simulink model "FCMW"  (R2024a)
settings: Solver=FixedStepAuto  StartTime=0.0  StopTime=inf  FixedStep=0.1
model workspace (MAT data in the model file):
  Ixx_values = 1.545e-05
  Iyy_values = 0.00073574
  Izz_values = 0.00074861
  base_link_Ixx = 7.46
  base_link_Iyy = 1.52
  base_link_Izz = 8.88
  base_link_mass = 19.0939
  gps0_Ixx = 2.1733e-06
  gps0_Iyy = 2.1733e-06
  gps0_Izz = 1.8e-07
  gps0_mass = 0.01
  i = 8
  imu_link_Ixx = 1e-05
  imu_link_Iyy = 1e-05
  imu_link_Izz = 1e-05
  imu_link_mass = 0.015
  masses = 0.085251
  phi = sym
  phi.s = 'symobj::fromString("eJytVL1OwzAQdpqWPwkhoaJCp0jwBIydCoKBEYoYWCyHmGLkOCXnlGbjKXgneCpst6LONQ0MjfTJzt35u+/uLIeEkBYhH59mbYdBxyzDPpl/odl3F3sTQ3YtoAQGIMbKmSv+c4t3LvIkmrJcsFjySLGUQ1QATyKhIijTLH69KtK0vEm40uJZ8Jz4OVuIs23xksnE2HteTL9mj/W6syAzjexbFqATKWKXe48sv30L4HpUphdSMOAwr/PEy/HtxQeIe9tiAoI+MFvY8MzTebo84/79vAcWc02DwfVskpmO4Vl8efFt9N9BfE6Hx+P7QgujEfOv1EF/J13xHVmsHeWSs1M7jyIGpP2wQYebFeVvBZPkr3429crn3LGATE65uwGV3jjfJQPxNOIa8fRQrKsn51ZZhd/hjlZ6gTV1US2+77hulkJpPnYdXs31uLlcrv6caZGp+rpu6eYejP9epKZHofniCJXw2UpeVyQ1iZkC6j0sliP0mhFEixXbgzX2+8X6AxDlhOk=", 2)'
  phi.Digits = 32
  rotors(1).mass = 0.085251
  rotors(1).Ixx = 1.545e-05
  rotors(1).Iyy = 0.00073574
  rotors(1).Izz = 0.00074861
  rotors(2).mass = 0.085251
  rotors(2).Ixx = 1.545e-05
  rotors(2).Iyy = 0.00073574
  rotors(2).Izz = 0.00074861
  rotors(3).mass = 0.085251
  rotors(3).Ixx = 1.545e-05
  rotors(3).Iyy = 0.00073574
  rotors(3).Izz = 0.00074861
  rotors(4).mass = 0.085251
  rotors(4).Ixx = 1.545e-05
  rotors(4).Iyy = 0.00073574
  rotors(4).Izz = 0.00074861
  rotors(5).mass = 0.085251
  rotors(5).Ixx = 1.545e-05
  rotors(5).Iyy = 0.00073574
  rotors(5).Izz = 0.00074861
  rotors(6).mass = 0.085251
  rotors(6).Ixx = 1.545e-05
  rotors(6).Iyy = 0.00073574
  rotors(6).Izz = 0.00074861
  rotors(7).mass = 0.085251
  rotors(7).Ixx = 1.545e-05
  rotors(7).Iyy = 0.00073574
  rotors(7).Izz = 0.00074861
  rotors(8).mass = 0.085251
  rotors(8).Ixx = 1.545e-05
  rotors(8).Iyy = 0.00073574
  rotors(8).Izz = 0.00074861
  theta = sym
  theta.s = 'symobj::fromString("eJytVL1OwzAQdpqWPwkhoaJCp0jwBIydCoKBESoxsFgOOYqR45ScU5qNp+CdylNhuxV13DQwNNInO3fn7767sxwSQlqEfH7ptR0GHb0M+2TxhXrfXe51DNk3wBIZIh9La674Lw0+gOdJNGU5Z7GASLIUMCoQkojLCMs0i99uijQt7xKQir9wyImbs+Vxtg1eM5Foe8+J6dfsfb32LIpMefYdA1SJ4LHNfUBW36EBghqV6ZXgDAEXdZ45Ob6d+MDj3jWYIKePzBQ2vHB0nq/O2H8375HBQtNgcDubZLpj/izmTnzb++94fFaHw+P6QgOt0edfq4P+TrriOzHYOMoVZ6d2HkWMnvbjBh12VhTeCybIX/1s6pXLuWeAmZiCvQGV3ljfNUP+PALl8fS8WFtPDkZZhd/igVZ64WvqerW4vtO6WXKpYGw7vJ7raXu5bP05UzyT9XXd0+09GP+9SE2PQvPF4TKB2VpeWyTViZlE6jwshiN0mhFEy9W3BxvssFx/ABFthPo=", 2)'
  theta.Digits = 32
  total_Ixx = 7.46
  total_Iyy = 1.53
  total_Izz = 8.89
  total_mass = 20
  total_rotor_Ixx = 0.0001236
  total_rotor_Iyy = 0.00588592
  total_rotor_Izz = 0.00598888
  total_rotor_masses = 0.682008
  u = sym
  u.s = 'symobj::fromString("eJytVL1OwzAQdpqWPwkhoaJCp0jwBIydCoKBESoxsFgOOYqR45ScU5qNp+CdylNhuxV13DQwNNInO3fn7767sxwSQlqEfH7ptR0GHb0M+2TxhXrfXe51DNk3wBIZIh9La674Lw0+gOdJNGU5Z7GASLIUMCoQkojLCMs0i99uijQt7xKQir9wyImbs+Vxtg1eM5Foe8+J6dfsfb32LIpMefYdA1SJ4LHNfUBW36EBghqV6ZXgDAEXdZ45Ob6d+MDj3jWYIKePzBQ2vHB0nq/O2H8375HBQtNgcDubZLpj/izmTnzb++94fFaHw+P6QgOt0edfq4P+TrriOzHYOMoVZ6d2HkWMnvbjBh12VhTeCybIX/1s6pXLuWeAmZiCvQGV3ljfNUP+PALl8fS8WFtPDkZZhd/igVZ64WvqerW4vtO6WXKpYGw7vJ7raXu5bP05UzyT9XXd0+09GP+9SE2PQvPF4TKB2VpeWyTViZlE6jwshiN0mhFEy9W3Bxvs0+X6AxH1hQs=", 2)'
  u.Digits = 32
  v = sym
  v.s = 'symobj::fromString("eJytVL1OwzAQdpqWPwkhoaJCp0jwBIydCoKBESoxsFgOOYqR45ScU5qNjTfgneCpsN2KOm4aGBrpk52783ff3VkOCSEtQt4/9doOg45ehn0y/0K97y72OobsGmCJDJGPpTVX/OcGb8DzJJqynLNYQCRZChgVCEnEZYRlmsUvV0WaljcJSMWfOOTEzdnyONsGz5lItL3nxPRr9r5eexZFpjz7lgGqRPDY5t4jy2/fAEGNyvRCcIaA8zpPnBzfTnzgcW8bTJDTe2YKG545Ok+XZ+y/m/fAYK5pMLieTTLdMX8WX0582/vveHxWh8Pj+kIDrdHnX6mD/k664jsyWDvKJWendh5FjJ72wwYddlYUXgsmyF/9bOqVy7ljgJmYgr0Bld5Y3yVD/jgC5fH0vFhbTw5GWYXf4o5WeuFr6nq1uL7jullyqWBsO7ya62FzuWz9OVM8k/V13dLNPRj/vUhNj0LzxeEygdlKXlsk1YmZROo8LIYjdJoRRIvVtwdr7B+L9QcSfYUc", 2)'
  v.Digits = 32
  w = sym
  w.s = 'symobj::fromString("eJytVL1OwzAQdpqWPwkhoaJCp0jwBIydCoKBESoxsFgOOYqR45ScU5qNp0C8EjwVtltRx00DQyN9snN3/u67O8shIaRFyPuHXtth0NHLsE/mX6j33cVex5BdAyyRIfKxtOaK/9zgDXieRFOWcxYLiCRLAaMCIYm4jLBMs/jlqkjT8iYBqfgTh5y4OVseZ9vgOROJtvecmH7N3tdrz6LIlGffMkCVCB7b3Htk+e0bIKhRmV4IzhBwXueJk+PbiQ887m2DCXJ6z0xhwzNH5+nyjP138x4YzDUNBtezSaY75s/iy4lve/8dj8/qcHhcX2igNfr8K3XQ30lXfEcGa0e55OzUzqOI0dN+2KDDzorCa8EE+aufTb1yOXcMMBNTsDeg0hvru2TIH0egPJ6eF2vrycEoq/Bb3NFKL3xNXa8W13dcN0suFYxth1dzPWwul60/Z4pnsr6uW7q5B+O/F6npUWi+OFwmMFvJa4ukOjGTSJ2HxXCETjOCaLH69mCN/XOx/gATBYUt", 2)'
  w.Digits = 32
  x = sym
  x.s = 'symobj::fromString("eJytVEtOwzAQdZqWn4SQUFGhq0hwApZdFQQLllCJBRvLIUMxcpyScUqz4xTcgaPAqbDdijpuGlg00pOdmfGbNzOWQ0JIi5D3D722w6Cjl2GfzL9Q77uLvY4huwZYIkPkY2nNFf+5wRvwPImmLOcsFhBJlgJGBUIScRlhmWbxy1WRpuVNAlLxJw45cXO2PM62wXMmEm3vOTH9mr2v155FkSnPvmWAKhE8trn3yPLbN0BQozK9EJwh4LzOEyfHtxMfeNzbBhPk9J6ZwoZnjs7T5Rn77+Y9MJhrGgyuZ5NMd8yfxZcT3/b+Ox6f1eHwuL7QQGv0+VfqoL+TrviODNaOcsnZqZ1HEaOn/bBBh50VhdeCCfJXP5t65XLuGGAmpmBvQKU31nfJkD+OQHk8PS/W1pODUVbht7ijlV74mrpeLa7vuG6WXCoY2w6v5nrYXC5bf84Uz2R9Xbd0cw/Gfy9S06PQfHG4TGC2ktcWSXViJpE6D4vhCJ1mBNFi9e3BGvvnYv0BE42FPg==", 2)'
  x.Digits = 32
  y = sym
  y.s = 'symobj::fromString("eJytVEtOwzAQdZqWn4SQUFGhq0hwApZdFQQLllCJBRvLIUMxcpyScUqz4xQchhvAqbDdijpuGlg00pOdmfGbNzOWQ0JIi5D3D722w6Cjl2GfzL9Q77uLvY4huwZYIkPkY2nNFf+5wRvwPImmLOcsFhBJlgJGBUIScRlhmWbxy1WRpuVNAlLxJw45cXO2PM62wXMmEm3vOTH9mr2v155FkSnPvmWAKhE8trn3yPLbN0BQozK9EJwh4LzOEyfHtxMfeNzbBhPk9J6ZwoZnjs7T5Rn77+Y9MJhrGgyuZ5NMd8yfxZcT3/b+Ox6f1eHwuL7QQGv0+VfqoL+TrviODNaOcsnZqZ1HEaOn/bBBh50VhdeCCfJXP5t65XLuGGAmpmBvQKU31nfJkD+OQHk8PS/W1pODUVbht7ijlV74mrpeLa7vuG6WXCoY2w6v5nrYXC5bf84Uz2R9Xbd0cw/Gfy9S06PQfHG4TGC2ktcWSXViJpE6D4vhCJ1mBNFi9e3BGvvnYv0BFBWFTw==", 2)'
  y.Digits = 32
  z = sym
  z.s = 'symobj::fromString("eJytVL1OwzAQdpqWPwkhoaJCp0jwBIydCoKBESoxsFgOOYqR45ScU5qNp+CdgJfCdivquGlgaKRPdu7O3313ZzkkhLQIef/QazsMOnoZ9sn8C/W+u9jrGLJrgCUyRD6W1lzxnxu8Ac+TaMpyzmIBkWQpYFQgJBGXEZZpFr9cFWla3iQgFX/ikBM3Z8vjbBs8ZyLR9p4T06/Z+3rtWRSZ8uxbBqgSwWObe48sv30DBDUq0wvBGQLO6zxxcnw58YHHvW0wQU7vmSlseOboPF2esf9u3gODuabB4Ho2yXTH/Fl8OvFt77/j8VkdDo/rCw20Rp9/pQ76O+mK78hg7SiXnJ3aeRQxetoPG3TYWVF4LZggf/WzqVcu544BZmIK9gZUemN9lwz54wiUx9PzYm09ORhlFX6LO1rpha+p69Xi+o7rZsmlgrHt8Gquh83lsvXnTPFM1td1Szf3YPz3IjU9Cs0Xh8sEZit5bZFUJ2YSqfOwGI7QaUYQLVbfHqyxfy/WHxSdhWA=", 2)'
  z.Digits = 32
undefined symbols (not defined in the file or in its folder): rad, s
libraries: robotlib x13, simulink x7, aerolibconvert2 x1, sharedtransform x1
settings Model: PacingRate=50  Creator=hmcl  LastModifiedBy=hmcl
settings OptimizationCC: EnhancedBackFolding=on  PassReuseOutputArgsAs=Individual arguments  ZeroExternalMemoryAtStartup=off  ZeroInternalMemoryAtStartup=off  MaxStackSize=64  OptimizeBlockOrder=speed  DifferentSizesBufferReuse=on  OptimizationCustomize=off  EfficientTunableParamExpr=on
settings DebuggingCC: ParameterTunabilityLossMsg=error
settings HardwareCC: ProdBitPerPointer=32  ProdBitPerSizeT=32  ProdBitPerPtrDiffT=32  ProdLargestAtomicFloat=None  ProdIntDivRoundTo=Undefined  ProdEndianess=Unspecified  ProdWordSize=32  ProdHWDeviceType=Generic->Unspecified (assume 32-bit Generic)
settings SFSimCC: MATLABDynamicMemAlloc=off
settings RTWCC: Description=Embedded Coder  SystemTargetFile=ert.tlc  HardwareBoard=Robot Operating System (ROS)  TLCOptions="-aInlineSetEventsForThisBaseRateFcn=TLC_FALSE -aSuppressMultiTaskScheduler=TLC_FALSE  -aRateBasedStepFcn=0"  TemplateMakefile=ert_default_tmf  Toolchain=Catkin  TargetLang=C++  GPUComputeCapability=3.5
settings CodeAppCC: ForceParamTrailComments=on  IgnoreCustomStorageClasses=off  OperatorAnnotations=on  SimulinkDataObjDesc=on  SFDataObjDesc=on  InsertBlockDesc=on
settings ERTTargetCC: ERTCustomFileTemplate=rostime_codertarget_file_process.tlc

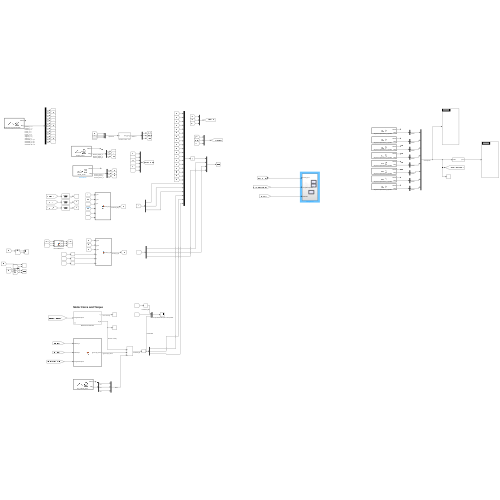
[thumbnail: Simulink's stored preview of the top-level diagram]
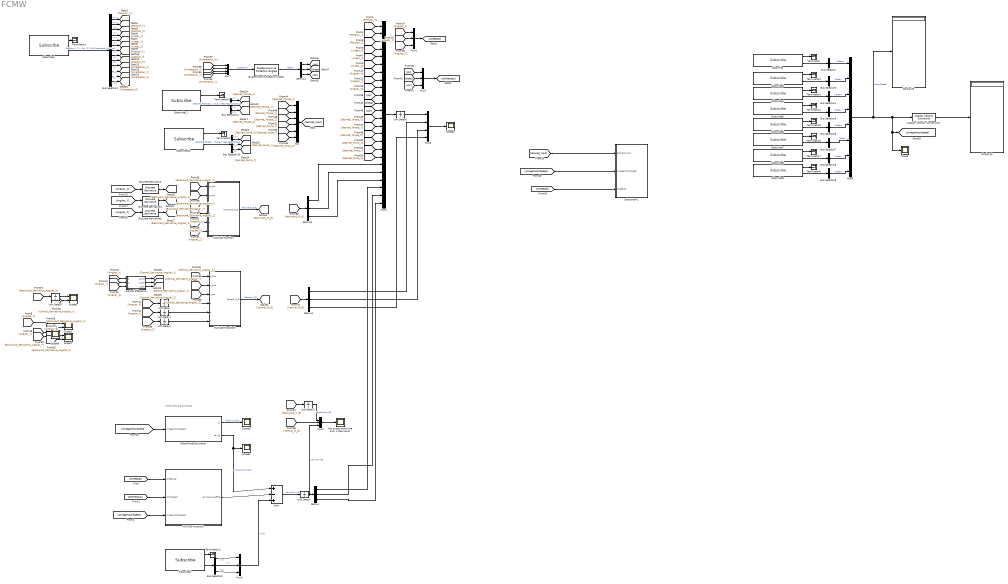
== system FCMW ==
  note: Motor Force and Torque
  Angular Velocity Conversion1 : aerolibconvert2/Angular Velocity Conversion  IU=rad/s  OU=rpm
  Bus Selector{,3..9} (8 alike) : BusSelector  OutputSignals=Data
  Bus Selector1 : BusSelector  OutputSignals=Pose.Pose.Position.X,Pose.Pose.Position.Y,Pose.Pose.Position.Z,Twist.Twist.Linear.X,Twist.Twist.Linear.Y,Twist.Twist.Linear.Z,Twist.Twist.Angular.X,Twist.Twist.Angular.Y,Twist.Twist.Angular.Z,Pose.Pose.Orientation.X,Pose.Pose.Orientation.Y,Pose.Pose.Orientation.Z,Pose.Pose.Orientation.W
  Bus Selector10 : BusSelector  OutputSignals=X,Y,Z
  Bus Selector11 : BusSelector  OutputSignals=X,Y,Z
  Bus Selector2 : BusSelector  OutputSignals=X,Y,Z
  Demux{,1,4..5} (4 alike) : Demux  Outputs=3
  Discrete Derivative : simulink/Discrete/Discrete Derivative  gainval=1  ICPrevScaledInput=0.0  OutMin=[]  OutMax=[]  OutDataType=fixdt(1, 16)  OutScaling=2^-10  DoSatur=off
  Discrete Derivative1 : simulink/Discrete/Discrete Derivative  gainval=1  ICPrevScaledInput=0.0  OutMin=[]  OutMax=[]  OutDataType=fixdt(1, 16)  OutScaling=2^-10  DoSatur=off
  Discrete Derivative2 : simulink/Discrete/Discrete Derivative  gainval=1  ICPrevScaledInput=0.0  OutMin=[]  OutMax=[]  OutDataType=fixdt(1, 16)  OutScaling=2^-10  DoSatur=off
  Display24 : Display
  Display25 : Display
  MATLAB Function : MATLAB Function  TreatAsAtomicUnit=on
  MATLAB Function1 : MATLAB Function  TreatAsAtomicUnit=on
  MATLAB Function3 : MATLAB Function  TreatAsAtomicUnit=on
  MotorForceCalculation : Subsystem  mask{b=0.00053, d=0.0000169, L1=0.545, L2=0.36, L3=1.08}
      mask prompts: b "b = motorConstant [N*s^2/rad^2] ="; d "d = momentConstant [N*m*s^2/rad^2] ="; L1 "L1 ="; L2 "L2 ="; L3 "L3 ="
  Mux : Mux  Inputs=6
  Mux{1..4} (4 alike) : Mux  Inputs=3
  Mux5 : Mux  Inputs=24
  Mux6 : Mux
  Mux7 : Mux
  Mux9 : Mux  Inputs=8
  Quaternions to Rotation Angles : sharedtransform/Quaternions to Rotation Angles  rotationOrder=ZYX  aMode=aMode
  Scope{,2..4} (4 alike) : Scope
  Scope{1,5..7} (4 alike) : Scope  NumInputPorts=2
  Subscribe : robotlib/Subscribe  topicSource=Select from ROS network  topic=/my/octocopter3/motor_speed/0  messageType=std_msgs/Float64  SampleTime=-1  legacyBusStruct=off  messageQueueLength=1
  Subscribe1 : robotlib/Subscribe  topicSource=Select from ROS network  topic=/mavros/local_position/odom  messageType=nav_msgs/Odometry  SampleTime=-1  legacyBusStruct=off  messageQueueLength=1
  Subscribe10 : robotlib/Subscribe  topicSource=Select from ROS network  topic=/thrust_vector  messageType=geometry_msgs/Vector3  SampleTime=-1  legacyBusStruct=off  messageQueueLength=1
  Subscribe11 : robotlib/Subscribe  topicSource=Select from ROS network  topic=/torque_vector  messageType=geometry_msgs/Vector3  SampleTime=-1  legacyBusStruct=off  messageQueueLength=1
  Subscribe2 : robotlib/Subscribe  topicSource=Select from ROS network  topic=/my_custom_wind  messageType=geometry_msgs/Vector3  SampleTime=-1  legacyBusStruct=off  messageQueueLength=1
  Subscribe3 : robotlib/Subscribe  topicSource=Select from ROS network  topic=/my/octocopter3/motor_speed/1  messageType=std_msgs/Float64  SampleTime=-1  legacyBusStruct=off  messageQueueLength=1
  Subscribe4 : robotlib/Subscribe  topicSource=Select from ROS network  topic=/my/octocopter3/motor_speed/2  messageType=std_msgs/Float64  SampleTime=-1  legacyBusStruct=off  messageQueueLength=1
  Subscribe5 : robotlib/Subscribe  topicSource=Select from ROS network  topic=/my/octocopter3/motor_speed/3  messageType=std_msgs/Float64  SampleTime=-1  legacyBusStruct=off  messageQueueLength=1
  Subscribe6 : robotlib/Subscribe  topicSource=Select from ROS network  topic=/my/octocopter3/motor_speed/4  messageType=std_msgs/Float64  SampleTime=-1  legacyBusStruct=off  messageQueueLength=1
  Subscribe7 : robotlib/Subscribe  topicSource=Select from ROS network  topic=/my/octocopter3/motor_speed/5  messageType=std_msgs/Float64  SampleTime=-1  legacyBusStruct=off  messageQueueLength=1
  Subscribe8 : robotlib/Subscribe  topicSource=Select from ROS network  topic=/my/octocopter3/motor_speed/6  messageType=std_msgs/Float64  SampleTime=-1  legacyBusStruct=off  messageQueueLength=1
  Subscribe9 : robotlib/Subscribe  topicSource=Select from ROS network  topic=/my/octocopter3/motor_speed/7  messageType=std_msgs/Float64  SampleTime=-1  legacyBusStruct=off  messageQueueLength=1
  Subsystem2 : Subsystem
  Sum : Sum  Inputs=|+-+
  Terminator{,1..11} (12 alike) : Terminator
  Unit Delay{,1..6} (7 alike) : UnitDelay  SampleTime=-1  HasFrameUpgradeWarning=on
  central difference : MATLAB Function  TreatAsAtomicUnit=on
  this scope shows the prior 1 step result : Scope
  wires:
  Mux7/1 -> Quaternions to Rotation Angles/1  "quertanion"
  Subscribe1/2 -> Bus Selector1/1  "Position_X = x  Position_Y = y Position_Z = z Linear_X = u Linear_Y = v Linear_Z = w Angular_X = p Angular_Y = q Angular_Z = r Orientation_X = q1  Orientation_Y = q2 Orientation_Z = q3 Orientation_W = q4"
  Subscribe1/1 -> Terminator1/1
  Subscribe/1 -> Terminator/1
  Subscribe3/1 -> Terminator2/1
  Subscribe4/1 -> Terminator3/1
  Subscribe5/1 -> Terminator4/1
  Subscribe6/1 -> Terminator5/1
  Subscribe7/1 -> Terminator6/1
  Subscribe8/1 -> Terminator7/1
  Subscribe9/1 -> Terminator8/1
  Subscribe/2 -> Bus Selector/1
  Subscribe3/2 -> Bus Selector3/1
  Subscribe4/2 -> Bus Selector4/1
  Subscribe5/2 -> Bus Selector5/1
  Subscribe6/2 -> Bus Selector6/1
  Subscribe7/2 -> Bus Selector7/1
  Subscribe8/2 -> Bus Selector8/1
  Subscribe9/2 -> Bus Selector9/1
  Mux9/1 -> Display25/1, Angular Velocity Conversion1/1, Scope/1, [omegaMotorSpeed]  "motorSpeed"
  Bus Selector/1 -> Mux9/1  "<Data>"
  Bus Selector3/1 -> Mux9/2  "<Data>"
  Bus Selector4/1 -> Mux9/3  "<Data>"
  Bus Selector5/1 -> Mux9/4  "<Data>"
  Bus Selector6/1 -> Mux9/5  "<Data>"
  Bus Selector7/1 -> Mux9/6  "<Data>"
  Bus Selector8/1 -> Mux9/7  "<Data>"
  Bus Selector9/1 -> Mux9/8  "<Data>"
  [desired_input] -> Subsystem2/1(desired_input)
  [omegaMotorSpeed] -> Subsystem2/2(omegaMotorSpeed)
  [OMEGAB] -> Subsystem2/3(OMEGAB)
  Angular Velocity Conversion1/1 -> Display24/1
  Mux5/1 -> Unit Delay6/1
  Subscribe10/1 -> Terminator9/1
  Subscribe11/1 -> Terminator10/1
  Subscribe10/2 -> Bus Selector10/1  "Desired_Force_X Desired_Force_Y Desired_Force_Z"
  Subscribe11/2 -> Bus Selector11/1  "Desired_Torque_X Desired_Torque_Y Desired_Torque_Z"
  Demux5/1 -> Mux5/19
  Demux5/2 -> Mux5/20
  Demux5/3 -> Mux5/21
  Mux/1 -> [desired_input]
  Mux1/1 -> [OMEGAB]
  [omegaMotorSpeed] -> MotorForceCalculation/1(omegaMotorSpeed)
  [OMEGAB] -> MATLAB Function1/1(OMEGA_B)
  Mux2/1 -> [phithetapsi]
  [phithetapsi] -> MATLAB Function1/2(phithetapsi)
  [omegaMotorSpeed] -> MATLAB Function1/3(omegaMotorSpeed)
  Subscribe2/1 -> Terminator11/1
  Subscribe2/2 -> Bus Selector2/1
  MATLAB Function1/1(gyroscopic_effect) -> Sum/2
  MotorForceCalculation/2(tau_B) -> Scope4/1, Sum/1  "moment on body"
  Bus Selector2/1 -> Mux3/1  "<X>"
  Bus Selector2/2 -> Mux3/2  "<Y>"
  Bus Selector2/3 -> Mux3/3  "<Z>"
  Mux3/1 -> Sum/3  "wind"
  MotorForceCalculation/1(f_t) -> Scope3/1  "force on body"
  Sum/1 -> Unit Delay4/1  "nominal M_B"
  Mux4/1 -> this scope shows the prior 1 step result/1
  Unit Delay/1 -> MATLAB Function3/4(p)
  Unit Delay1/1 -> MATLAB Function3/5(q)
  Unit Delay2/1 -> MATLAB Function3/6(r)
  Unit Delay3/1 -> Mux4/1  "backward_MB"
  Unit Delay5/1 -> Scope5/1
  Unit Delay4/1 -> Mux4/3, Demux/1  "nominal MB"
  Demux/1 -> Mux5/22
  Demux/2 -> Mux5/23
  Demux/3 -> Mux5/24
  Unit Delay6/1 -> Mux6/1
  Mux6/1 -> Scope2/1
  Demux1/1 -> Mux6/2
  Demux1/2 -> Mux6/3
  Demux1/3 -> Mux6/4
  Bus Selector1/1 -> [Position_X]  "<X>"
  [Position_X] -> Mux5/1
  Bus Selector1/2 -> [Position_Y]  "<Y>"
  [Position_Y] -> Mux5/2
  Bus Selector1/3 -> [Position_Z]  "<Z>"
  [Position_Z] -> Mux5/3
  Bus Selector1/4 -> [Linear_X]  "<X>"
  [Linear_X] -> Mux5/4
  Bus Selector1/5 -> [Linear_Y]  "<Y>"
  [Linear_Y] -> Mux5/5
  Bus Selector1/6 -> [Linear_Z]  "<Z>"
  [Linear_Z] -> Mux5/6
  Bus Selector1/7 -> [Angular_X]  "<X>"
  [Angular_X] -> Scope1/1
  [Angular_X] -> central difference/1(p)
  [Angular_X] -> Unit Delay/1
  [Angular_X] -> Mux5/7
  [Angular_X] -> Mux1/1
  [Angular_X] -> Discrete Derivative/1
  [Angular_X] -> MATLAB Function/4(p)
  Bus Selector1/8 -> [Angular_Y]  "<Y>"
  [Angular_Y] -> Discrete Derivative1/1
  [Angular_Y] -> Scope6/1
  [Angular_Y] -> MATLAB Function/5(q)
  [Angular_Y] -> Unit Delay1/1
  [Angular_Y] -> Mux5/8
  [Angular_Y] -> Mux1/2
  [Angular_Y] -> central difference/2(q)
  Bus Selector1/9 -> [Angular_Z]  "<Z>"
  [Angular_Z] -> Mux1/3
  [Angular_Z] -> Discrete Derivative2/1
  [Angular_Z] -> Scope7/1
  [Angular_Z] -> Mux5/9
  [Angular_Z] -> MATLAB Function/6(r)
  [Angular_Z] -> central difference/3(r)
  [Angular_Z] -> Unit Delay2/1
  Bus Selector1/10 -> [Orientation_X]  "<X>"
  [Orientation_X] -> Mux7/4
  Bus Selector1/11 -> [Orientation_Y]  "<Y>"
  [Orientation_Y] -> Mux7/3
  Bus Selector1/12 -> [Orientation_Z]  "<Z>"
  [Orientation_Z] -> Mux7/2
  Bus Selector1/13 -> [Orientation_W]  "<W>"
  [Orientation_W] -> Mux7/1
  Quaternions to Rotation Angles/1 -> Demux4/1  "radian"
  Demux4/1 -> [phi]
  [phi] -> Mux5/10
  [phi] -> Mux2/1
  Demux4/2 -> [theta]
  [theta] -> Mux5/11
  [theta] -> Mux2/2
  Demux4/3 -> [psi]
  [psi] -> Mux2/3
  [psi] -> Mux5/12
  Bus Selector11/1 -> [Desired_Torque_X]  "<X>"
  [Desired_Torque_X] -> Mux/1
  [Desired_Torque_X] -> Mux5/13
  Bus Selector11/2 -> [Desired_Torque_Y]  "<Y>"
  [Desired_Torque_Y] -> Mux/2
  [Desired_Torque_Y] -> Mux5/14
  Bus Selector11/3 -> [Desired_Torque_Z]  "<Z>"
  [Desired_Torque_Z] -> Mux/3
  [Desired_Torque_Z] -> Mux5/15
  Bus Selector10/1 -> [Desired_Force_X]  "<X>"
  [Desired_Force_X] -> Mux5/16
  [Desired_Force_X] -> Mux/4
  Bus Selector10/2 -> [Desired_Force_Y]  "<Y>"
  [Desired_Force_Y] -> Mux5/17
  [Desired_Force_Y] -> Mux/5
  Bus Selector10/3 -> [Desired_Force_Z]  "<Z>"
  [Desired_Force_Z] -> Mux5/18
  [Desired_Force_Z] -> Mux/6
  Discrete Derivative/1 -> [Backward_Derivative_Angular_X]
  [Backward_Derivative_Angular_X] -> MATLAB Function/1(p_dot)
  [Backward_Derivative_Angular_X] -> Unit Delay5/1
  [Backward_Derivative_Angular_X] -> Scope1/2
  Discrete Derivative1/1 -> [Backward_Derivative_Angular_Y]
  [Backward_Derivative_Angular_Y] -> MATLAB Function/2(q_dot)
  [Backward_Derivative_Angular_Y] -> Scope6/2
  Discrete Derivative2/1 -> [Backward_Derivative_Angular_Z]
  [Backward_Derivative_Angular_Z] -> MATLAB Function/3(r_dot)
  [Backward_Derivative_Angular_Z] -> Scope7/2
  central difference/1(p_dot) -> [Central_Derivative_Angular_X]
  [Central_Derivative_Angular_X] -> Scope5/2
  [Central_Derivative_Angular_X] -> MATLAB Function3/1(p_dot)
  central difference/2(q_dot) -> [Central_Derivative_Angular_Y]
  [Central_Derivative_Angular_Y] -> MATLAB Function3/2(q_dot)
  central difference/3(r_dot) -> [Central_Derivative_Angular_Z]
  [Central_Derivative_Angular_Z] -> MATLAB Function3/3(r_dot)
  MATLAB Function/1(backward_M_B) -> [backward_M_B]  "backward_M_B"
  [backward_M_B] -> Unit Delay3/1
  [backward_M_B] -> Demux5/1
  MATLAB Function3/1(Central_M_B) -> [Central_M_B]  "Central_M_B"
  [Central_M_B] -> Mux4/2
  [Central_M_B] -> Demux1/1

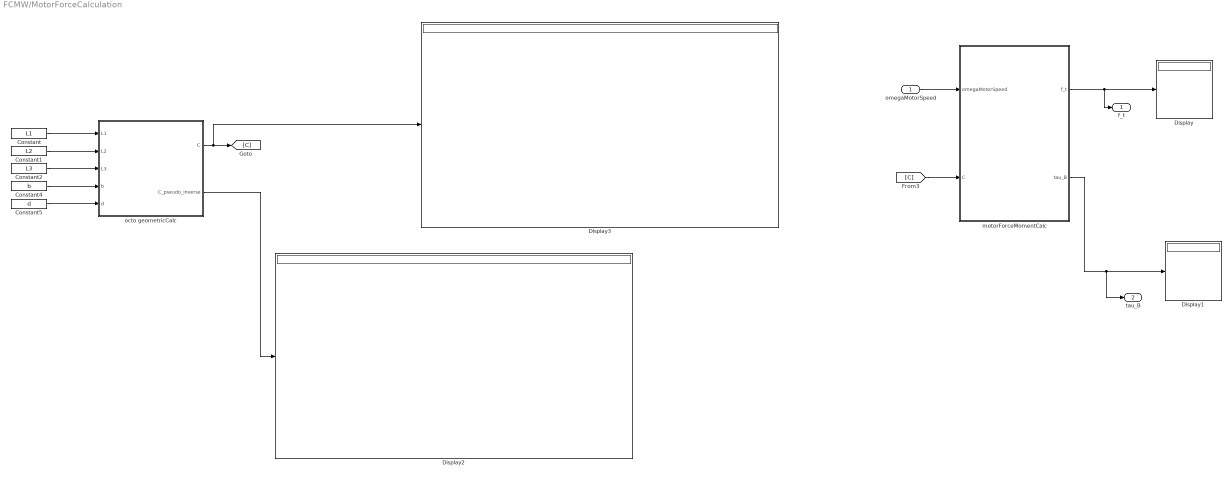
== system FCMW/MotorForceCalculation ==
  omegaMotorSpeed : Inport
  Constant : Constant  Value=L1
  Constant1 : Constant  Value=L2
  Constant2 : Constant  Value=L3
  Constant4 : Constant  Value=b
  Constant5 : Constant  Value=d
  Display{,1..3} (4 alike) : Display
  motorForceMomentCalc : MATLAB Function  TreatAsAtomicUnit=on
  octo geometricCalc : MATLAB Function  TreatAsAtomicUnit=on
  f_t : Outport
  tau_B : Outport  Port=2
  wires:
  motorForceMomentCalc/1(f_t) -> f_t/1, Display/1
  motorForceMomentCalc/2(tau_B) -> tau_B/1, Display1/1
  [C] -> motorForceMomentCalc/2(C)
  Constant2/1 -> octo geometricCalc/3(L3)
  Constant5/1 -> octo geometricCalc/5(d)
  Constant/1 -> octo geometricCalc/1(L1)
  Constant4/1 -> octo geometricCalc/4(b)
  octo geometricCalc/1(C) -> [C], Display3/1
  Constant1/1 -> octo geometricCalc/2(L2)
  octo geometricCalc/2(C_pseudo_inverse) -> Display2/1
  omegaMotorSpeed/1 -> motorForceMomentCalc/1(omegaMotorSpeed)

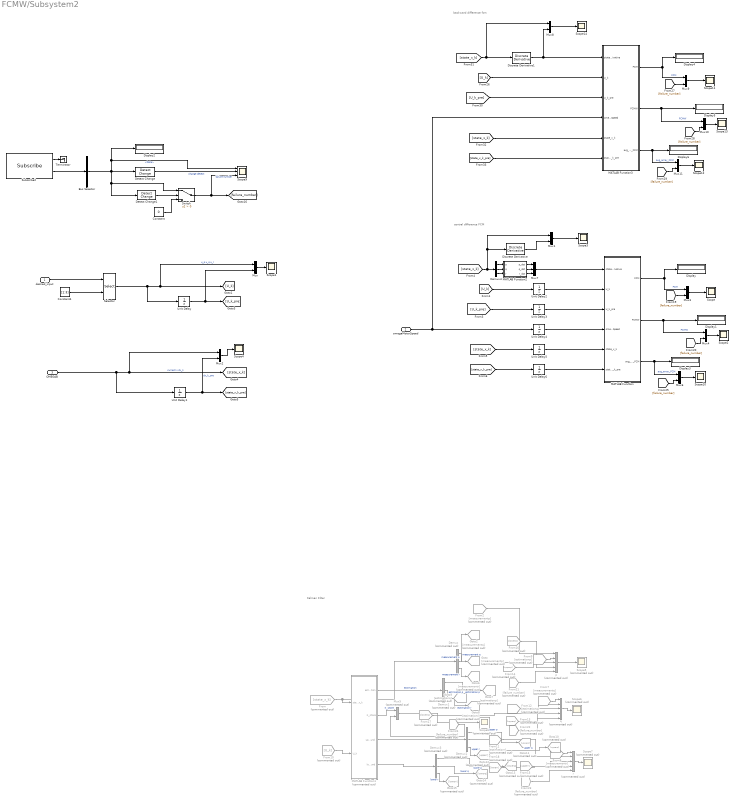
== system FCMW/Subsystem2 ==
  note: Kalman Filter
  note: backward difference fcm
  note: central difference FCM
  desired_input : Inport
  omegaMotorSpeed : Inport  Port=2
  OMEGAB : Inport  Port=3
  Bus Selector : BusSelector  OutputSignals=Data
  Constant : Constant  Value=0
  Constant4 : Constant  Value=[1:3]
  Demux{,1..3} (4 alike) : Demux  Commented=on  Outputs=3
  Demux4 : Demux  Outputs=3
  Detect Change : simulink/Logic and Bit Operations/Detect Change  vinit=0  OutDataTypeStr=boolean
  Detect Change1 : simulink/Logic and Bit Operations/Detect Change  vinit=0  OutDataTypeStr=boolean
  Discrete Derivative : simulink/Discrete/Discrete Derivative  gainval=0.5  ICPrevScaledInput=0.0  OutMin=[]  OutMax=[]  OutDataType=fixdt(1, 16)  OutScaling=2^-10  DoSatur=off
  Discrete Derivative1 : simulink/Discrete/Discrete Derivative  gainval=0.5  ICPrevScaledInput=0.0  OutMin=[]  OutMax=[]  OutDataType=fixdt(1, 16)  OutScaling=2^-10  DoSatur=off
  Display{,1..6} (7 alike) : Display
  From : From  Commented=on  GotoTag=state_x_k
  From10 : From  Commented=on  GotoTag=U_k
  From11 : From  Commented=on  GotoTag=estimationr
  From12 : From  Commented=on  GotoTag=estimationq
  From13 : From  Commented=on  GotoTag=upperq
  From14 : From  Commented=on  GotoTag=upperp
  From15 : From  Commented=on  GotoTag=upperr
  From16 : From  Commented=on  GotoTag=lowerp
  From17 : From  Commented=on  GotoTag=lowerq
  From18 : From  Commented=on  GotoTag=lowerr
  From2 : From  Commented=on  GotoTag=measurementp
  From{21..24} (4 alike) : From  Commented=on  GotoTag=failure_number
  From7 : From  Commented=on  GotoTag=measurementq
  From8 : From  Commented=on  GotoTag=measurementr
  From9 : From  Commented=on  GotoTag=estimationp
  Goto : Goto  Commented=on  GotoTag=measurementp
  Goto10 : Goto  Commented=on  GotoTag=upperq
  Goto11 : Goto  Commented=on  GotoTag=upperp
  Goto12 : Goto  Commented=on  GotoTag=upperr
  Goto13 : Goto  Commented=on  GotoTag=lowerp
  Goto14 : Goto  Commented=on  GotoTag=lowerq
  Goto15 : Goto  Commented=on  GotoTag=lowerr
  Goto2 : Goto  Commented=on  GotoTag=measurementq
  Goto6 : Goto  Commented=on  GotoTag=measurementr
  Goto7 : Goto  Commented=on  GotoTag=estimationp
  Goto8 : Goto  Commented=on  GotoTag=estimationr
  Goto9 : Goto  Commented=on  GotoTag=estimationq
  MATLAB Function : MATLAB Function  TreatAsAtomicUnit=on
  MATLAB Function1 : MATLAB Function  Commented=on  TreatAsAtomicUnit=on
  MATLAB Function2 : MATLAB Function  TreatAsAtomicUnit=on
  MATLAB Function3 : MATLAB Function  TreatAsAtomicUnit=on
  Mux{,1..4,6,8..11} (10 alike) : Mux  Inputs=2
  Mux5 : Mux  Commented=on  Inputs=2
  Mux7 : Mux  Inputs=3
  Scope{,1..4,10..14} (10 alike) : Scope
  Scope{5..8} (4 alike) : Scope  Commented=on
  Scope9 : Scope  NumInputPorts=3
  Selector : Selector  InputPortWidth=6  IndexOptions=Index vector (port)  Indices=[1 3]  OutputSizes=1
  Subscribe2 : robotlib/Subscribe  topicSource=Select from ROS network  topic=/mavros/keyboard_command/keyboard_float  messageType=std_msgs/Float32  SampleTime=-1  legacyBusStruct=off  messageQueueLength=1
  Switch : Switch  Criteria=u2 > Threshold  SaturateOnIntegerOverflow=off  InputSameDT=off
  Terminator : Terminator
  Unit Delay{,1..6} (7 alike) : UnitDelay  SampleTime=-1  HasFrameUpgradeWarning=on
  p : Mux  Commented=on  Inputs=5
  q : Mux  Commented=on  Inputs=5
  r : Mux  Commented=on  Inputs=5
  wires:
  desired_input/1 -> Selector/1
  Unit Delay/1 -> Mux/2, [U_k_pre]
  OMEGAB/1 -> Mux2/1, [state_x_k], Unit Delay1/1  "current x dx_k"
  Unit Delay1/1 -> Mux2/2, [state_x_k_pre]  "dx_k_pre"
  Constant4/1 -> Selector/2
  Selector/1 -> Mux/1, [U_k], Unit Delay/1  "u_p u_q u_r"
  Mux/1 -> Scope1/1
  Mux2/1 -> Scope4/1
  Subscribe2/1 -> Terminator/1
  Subscribe2/2 -> Bus Selector/1
  Bus Selector/1 -> Switch/1, Detect Change1/1, Scope9/1, Display2/1, Detect Change/1  "<Data>"
  Detect Change/1 -> Scope9/2  "change detect"
  Detect Change1/1 -> Switch/2
  Switch/1 -> [failure_number], Scope9/3  "failure number"
  Constant/1 -> Switch/3
  MATLAB Function/1(FCM) -> Mux3/1, Display/1  "FCM"
  [failure_number] -> Mux4/2
  [state_x_k_pre] -> Unit Delay6/1
  [state_x_k] -> Demux4/1, Mux1/1, Discrete Derivative/1
  Unit Delay3/1 -> MATLAB Function/3(U_k_pre)
  [failure_number] -> Mux6/2
  Mux1/1 -> Scope3/1
  Unit Delay6/1 -> MATLAB Function/6(state_x_k_pre)
  [U_k] -> Unit Delay2/1
  MATLAB Function/3(avg_array_FCM) -> Mux6/1, Display3/1  "avg_array_FCM"
  Discrete Derivative/1 -> Mux1/2
  Unit Delay4/1 -> MATLAB Function/4(omegaMotorSpeed)
  Mux7/1 -> MATLAB Function/1(state_derivative)
  Mux6/1 -> Scope10/1
  MATLAB Function/2(FCMW) -> Mux4/1, Display1/1  "FCMW"
  Demux4/3 -> MATLAB Function2/3(r)
  MATLAB Function2/2(q_dot) -> Mux7/2
  Mux3/1 -> Scope/1
  Unit Delay2/1 -> MATLAB Function/2(U_k)
  [failure_number] -> Mux3/2
  MATLAB Function2/3(r_dot) -> Mux7/3
  Mux4/1 -> Scope2/1
  [state_x_k] -> Unit Delay5/1
  Demux4/1 -> MATLAB Function2/1(p)
  Demux4/2 -> MATLAB Function2/2(q)
  Unit Delay5/1 -> MATLAB Function/5(state_x_k)
  MATLAB Function2/1(p_dot) -> Mux7/1
  [U_k_pre] -> Unit Delay3/1
  [failure_number] -> Mux9/2
  Mux11/1 -> Scope12/1
  MATLAB Function3/2(FCMW) -> Mux10/1, Display5/1  "FCMW"
  Discrete Derivative1/1 -> MATLAB Function3/1(state_derivative), Mux8/2
  [state_x_k] -> Mux8/1, Discrete Derivative1/1
  [U_k_pre] -> MATLAB Function3/3(U_k_pre)
  Mux10/1 -> Scope13/1
  [state_x_k] -> MATLAB Function3/5(state_x_k)
  [failure_number] -> Mux10/2
  Mux9/1 -> Scope11/1
  MATLAB Function3/3(avg_array_FCM) -> Mux11/1, Display6/1  "avg_array_FCM"
  Mux8/1 -> Scope14/1
  [failure_number] -> Mux11/2
  MATLAB Function3/1(FCM) -> Mux9/1, Display4/1  "FCM"
  [U_k] -> MATLAB Function3/2(U_k)
  omegaMotorSpeed/1 -> MATLAB Function3/4(omegaMotorSpeed), Unit Delay4/1
  [state_x_k_pre] -> MATLAB Function3/6(state_x_k_pre)
  Demux1/3 -> Goto8/1  "estimation r"
  MATLAB Function1/1(estimation) -> Demux1/1  "estimation"
  MATLAB Function1/4(lower_bound) -> Demux3/1
  From2/1 -> p/1
  From13/1 -> q/3
  From21/1 -> p/5
  From12/1 -> q/2
  From16/1 -> p/4
  Demux/1 -> Goto/1  "measurement p"
  Demux1/2 -> Goto9/1  "estimation q"
  Demux3/2 -> Goto14/1  "lower q"
  q/1 -> Scope6/1
  From18/1 -> r/4
  Demux1/1 -> Goto7/1  "estimation p"
  r/1 -> Scope7/1
  From23/1 -> r/5
  Demux/2 -> Goto2/1  "measurement q"
  Demux2/2 -> Goto10/1  "upper q"
  From9/1 -> p/2
  From/1 -> Demux/1, MATLAB Function1/1(state_x_k)
  From14/1 -> p/3
  Demux3/3 -> Goto15/1  "lower r"
  Demux3/1 -> Goto13/1  "lower p"
  Demux2/1 -> Goto11/1  "upper p"
  From22/1 -> q/5
  From10/1 -> MATLAB Function1/2(U_k)
  From11/1 -> r/2
  From24/1 -> Mux5/2
  From7/1 -> q/1
  p/1 -> Scope5/1
  From17/1 -> q/4
  MATLAB Function1/3(upper_bound) -> Demux2/1
  Demux/3 -> Goto6/1  "measurement r"
  MATLAB Function1/2(K_store) -> Mux5/1  "K_store"
  From15/1 -> r/3
  Mux5/1 -> Scope8/1
  From8/1 -> r/1
  Demux2/3 -> Goto12/1  "upper r"

== matlab function FCMW/Subsystem2/MATLAB Function2 ==
  data: p input; p_dot output; q input; r input; q_dot output; r_dot output
function [p_dot, q_dot, r_dot] = fcn(p, q, r)
    % 중앙 차분법으로 p_dot, q_dot, r_dot 계산
    % 그런데 중앙차분할때 미래의 데이터를 알아야하는데 알수가 없기 때문에 여기서 얻는 중앙차분값은 한스텦 이전의 상태에서의 미분값이다.

    % 상태 유지 변수
    persistent data_p data_q data_r dt initialized;

    % 초기화
    if isempty(initialized)
        data_p = zeros(3, 1); % 고정된 크기의 배열
        data_q = zeros(3, 1);
        data_r = zeros(3, 1);
        dt = 0.1; % 샘플링 간격
        initialized = true;
    end

    % FIFO 방식으로 데이터 업데이트
    data_p = [data_p(2:end); p]; % 가장 오래된 데이터 제거 후 새로운 데이터 추가
    data_q = [data_q(2:end); q];
    data_r = [data_r(2:end); r];

    % 중앙 차분법 적용 (배열 크기가 3인 경우)
    p_dot = (data_p(3) - data_p(1)) / (2 * dt); % 중앙 차분
    q_dot = (data_q(3) - data_q(1)) / (2 * dt); % 중앙 차분
    r_dot = (data_r(3) - data_r(1)) / (2 * dt); % 중앙 차분

    disp("data_p = ");
    disp(data_p);
end

== matlab function FCMW/Subsystem2/MATLAB Function3 ==
  settings: updateMethod=DISCRETE
  data: state_derivative input; U_k input; U_k_pre input; FCM output; omegaMotorSpeed input; state_x_k input; state_x_k_pre input; FCMW output; avg_array_FCM output
function [FCM, FCMW, avg_array_FCM]  = fcn(state_derivative,U_k,U_k_pre,omegaMotorSpeed,state_x_k,state_x_k_pre)


% X_k = current
% X_k_pre = previous


coder.extrinsic('delft_evaluate_jacobians');
coder.extrinsic('size');
coder.extrinsic('ctrb');
coder.extrinsic('rank');
coder.extrinsic('inv');
coder.extrinsic('sign');
coder.extrinsic('calculate_FCMW');
coder.extrinsic('diff');
% persistent 변수 선언
persistent initialized avg_array_FCM_;

dt = 0.004; % 시간 간격 % 가제보는 dt = 0.004 로 데이터를 전송및 한다
omega_max = 425.47; % 최대 회전 속도 rad/s, maxRotVelocity in sdf
tau = 0.01; % 액추에이터 시간 상수
M = eye(3);
window_size_ = 50;

delft_df_dx = zeros(length(state_x_k), length(state_x_k));
delft_df_du = zeros(length(state_x_k), length(U_k));
del_umax = zeros(3,1);
del_uc = zeros(3,1);
signMask = zeros(1,8);
refOmega = zeros(8,1);
signError = zeros(1,1);
rank_con = 0;

rotorMapping = [1 -1 1;
    -1 1 1;
    1 -1 -1;
    1 1 -1;
    -1 -1 -1;
    -1 1 -1;
    -1 -1 1;
    1 1 1];

% rotorMapping = rotorMapping *-1; 

% x = state_x_k1(1);
% y = state_x_k1(2);
% z = state_x_k1(3);
% u = state_x_k1(4);
% v = state_x_k1(5);
% w = state_x_k1(6);
% phi = state_x_k1(7);
% theta = state_x_k1(8);
% psi = state_x_k1(9);
p = state_x_k(1);
q = state_x_k(2);
r = state_x_k(3);

u_p = U_k(1);
u_q = U_k(2);
u_r = U_k(3);



% 초기화가 필요할 때만 실행
if isempty(initialized)
    initialized = true; % 초기화 완료 표시
    FCMW = 1;
    avg_array_FCM = 1.0;
    avg_array_FCM_ = 1.0;
    disp('initialized.');
end

disp('-----------------');
% 심볼릭 야코비안 행렬 평가
[df_dx_temp, df_du_temp] = delft_evaluate_jacobians(p, q, r, u_p, u_q, u_r);

% 외부 함수로부터 받은 값을 MATLAB 배열로 변환
delft_df_dx = df_dx_temp; %delft_df_dx = A %3by3   %length(X_k1) by length(X_k1)

delft_df_du = df_du_temp; %delft_df_du = B %3by3    %length(X_k1) by length(U_k1)

A = delft_df_dx;
B = delft_df_du;

% 상태 및 입력 차이 계산
dx = state_x_k - state_x_k_pre;  % dx는 3x1
du = U_k - U_k_pre;  % du는 3x1



% disp('size(delft_df_dx) = ')
% disp(size(delft_df_dx))
% disp('B = ')
% disp(B)

% dx_dot = df_dx * dx + df_du * du;
%{
state X 가 정확값이라고 했을때 state X를 미분하면 dx_dot 이 나오게 된다.
그리고 식(6)을 보면 dx_dot 을 근사한 식인 A * dx + B * du 가 있다.
만약 근사한식이 너무 정확하면 dx_dot - (A * dx + B * du) 을 했을때 0 이 된다.
즉, 근사한 식이 정확하면 미분한 식(dx_dot) - 근사한식(A * dx + B * du) 이 0이 되야한다.

하지만 근사한식이 당연히 정확할수 없기 때문에 error가 생기는데
이 에러를 보상해주기 위해, 또는 0으로 수렴 시키기 위해서
del_uc를 정의 해준다.
del_uc는 inv(B) *error 이다.

그래서 dx_dot - (A * dx + B * du + del_uc) 식(11)이 나오고 이 식은 0으로 점점 수렴하게 된다.
%}

corrcoef_result = corrcoef(state_derivative, A * dx + B * du);

for i = 1:3
    if ~isnan(corrcoef_result(1,2))
        M(i, i) = max(corrcoef_result(1,2), 0.001); % 최소값 설정
    else
        M(i, i) = 0.001; % NaN일 경우 기본값 설정
    end
end

% disp('Updated M matrix:');
% disp(M);

B = B * M;

% disp('B = ')
% disp(B)

disp('state_derivative = ');
disp(state_derivative);

disp('A * dx + B * du = ');
disp(A * dx + B * du);

error = state_derivative - (A * dx + B * du); %error : 3by1
disp('error = ');
disp(error);

if (error == 0)
    
    disp('error is zero');
    FCM = 1;
    FCMW = 1;
    avg_array_FCM = avg_array_FCM_;
    return

else
    del_uc = (inv(B)) * error; % del_uc는 3x1


    rotorMapping = rotorMapping'; % 이건 필수인듯?
    % disp('rotorMapping = ')
    % disp(rotorMapping(1,:))



    % error의 부호를 계산
    for i = 1:length(error)

        signError = sign(error(i));
        % disp('signError = ')
        % disp(signError)

        signMask = signError .* rotorMapping(i,:); % sign(error)를 대체
        % disp('signMask = ')
        % disp(signMask)

        for j = 1:length(signMask)
            if signMask(j) < 0
                refOmega(j) = omega_max; % signMask가 0보다 작으면 omega_max 할당
            else
                refOmega(j) = 0;         % signMask가 0 이상이면 0 할당
            end
        end

        % disp('refOmega = ');
        % disp(refOmega);

        % disp('omegaMotorSpeed = ');
        % disp(omegaMotorSpeed);

        maxDiff = abs(abs(omegaMotorSpeed) - refOmega); %maxDiff  8by1
        % disp('maxDiff = ')
        % disp(maxDiff)

        % Δu_MAX
        del_umax(i,1) = dt * (1/tau) * sum(maxDiff);
    end


    disp('abs(del_uc) = ')
    disp(abs(del_uc))

    disp('del_umax = ');
    disp(del_umax);


    controllability_matrix = ctrb(A,B);
    % disp('controllability_matrix = ')
    % disp(controllability_matrix)

    % 랭크 계산
    rank_con = rank(controllability_matrix);


    % disp('rank_con = ');
    % disp(rank_con);

    n = length(A);

    % disp('n = ')
    % disp(size(n))

    if rank_con < n || any(del_umax < abs(del_uc))
        FCM = 0;
    else
        FCM = 1;
    end

    [FCMW_, avg_array_FCM_] = calculate_FCMW(FCM,window_size_);

    FCMW = FCMW_;
    avg_array_FCM = avg_array_FCM_;

end % if end

disp('-----------------');

end

== matlab function FCMW/MATLAB Function ==
  data: backward_M_B output; p_dot input; q_dot input; r_dot input; p input; q input; r input
function backward_M_B = fcn(p_dot,q_dot,r_dot,p,q,r)


I_v = [7.46 0 0;0 1.53 0;0 0 8.89];

backward_M_B = I_v * [p_dot;q_dot;r_dot] + cross([p;q;r] , I_v * [p;q;r]);

== matlab function FCMW/Subsystem2/MATLAB Function ==
  settings: updateMethod=DISCRETE
  data: state_derivative input; U_k input; U_k_pre input; FCM output; omegaMotorSpeed input; state_x_k input; state_x_k_pre input; FCMW output; avg_array_FCM output
function [FCM, FCMW, avg_array_FCM]  = fcn(state_derivative,U_k,U_k_pre,omegaMotorSpeed,state_x_k,state_x_k_pre)


% X_k = current
% X_k_pre = previous


coder.extrinsic('delft_evaluate_jacobians');
coder.extrinsic('size');
coder.extrinsic('ctrb');
coder.extrinsic('rank');
coder.extrinsic('inv');
coder.extrinsic('sign');
coder.extrinsic('calculate_FCMW');
coder.extrinsic('diff');
% persistent 변수 선언
persistent initialized avg_array_FCM_;

dt = 0.004; % 시간 간격 % 가제보는 dt = 0.004 로 데이터를 전송및 한다
omega_max = 425.47; % 최대 회전 속도 rad/s, maxRotVelocity in sdf
tau = 0.01; % 액추에이터 시간 상수
M = eye(3);
window_size_ = 50;

delft_df_dx = zeros(length(state_x_k), length(state_x_k));
delft_df_du = zeros(length(state_x_k), length(U_k));
del_umax = zeros(3,1);
del_uc = zeros(3,1);
signMask = zeros(1,8);
refOmega = zeros(8,1);
signError = zeros(1,1);
rank_con = 0;

rotorMapping = [1 -1 1;
    -1 1 1;
    1 -1 -1;
    1 1 -1;
    -1 -1 -1;
    -1 1 -1;
    -1 -1 1;
    1 1 1];

% rotorMapping = rotorMapping *-1; 

% x = state_x_k1(1);
% y = state_x_k1(2);
% z = state_x_k1(3);
% u = state_x_k1(4);
% v = state_x_k1(5);
% w = state_x_k1(6);
% phi = state_x_k1(7);
% theta = state_x_k1(8);
% psi = state_x_k1(9);
p = state_x_k(1);
q = state_x_k(2);
r = state_x_k(3);

u_p = U_k(1);
u_q = U_k(2);
u_r = U_k(3);



% 초기화가 필요할 때만 실행
if isempty(initialized)
    initialized = true; % 초기화 완료 표시
    FCMW = 1;
    avg_array_FCM = 1.0;
    avg_array_FCM_ = 1.0;
    disp('initialized.');
end

disp('-----------------');
% 심볼릭 야코비안 행렬 평가
[df_dx_temp, df_du_temp] = delft_evaluate_jacobians(p, q, r, u_p, u_q, u_r);

% 외부 함수로부터 받은 값을 MATLAB 배열로 변환
delft_df_dx = df_dx_temp; %delft_df_dx = A %3by3   %length(X_k1) by length(X_k1)

delft_df_du = df_du_temp; %delft_df_du = B %3by3    %length(X_k1) by length(U_k1)

A = delft_df_dx;
B = delft_df_du;

% 상태 및 입력 차이 계산
dx = state_x_k - state_x_k_pre;  % dx는 3x1
du = U_k - U_k_pre;  % du는 3x1



% disp('size(delft_df_dx) = ')
% disp(size(delft_df_dx))
% disp('B = ')
% disp(B)

% dx_dot = df_dx * dx + df_du * du;
%{
state X 가 정확값이라고 했을때 state X를 미분하면 dx_dot 이 나오게 된다.
그리고 식(6)을 보면 dx_dot 을 근사한 식인 A * dx + B * du 가 있다.
만약 근사한식이 너무 정확하면 dx_dot - (A * dx + B * du) 을 했을때 0 이 된다.
즉, 근사한 식이 정확하면 미분한 식(dx_dot) - 근사한식(A * dx + B * du) 이 0이 되야한다.

하지만 근사한식이 당연히 정확할수 없기 때문에 error가 생기는데
이 에러를 보상해주기 위해, 또는 0으로 수렴 시키기 위해서
del_uc를 정의 해준다.
del_uc는 inv(B) *error 이다.

그래서 dx_dot - (A * dx + B * du + del_uc) 식(11)이 나오고 이 식은 0으로 점점 수렴하게 된다.
%}

corrcoef_result = corrcoef(state_derivative, A * dx + B * du);

for i = 1:3
    if ~isnan(corrcoef_result(1,2))
        M(i, i) = max(corrcoef_result(1,2), 0.001); % 최소값 설정
    else
        M(i, i) = 0.001; % NaN일 경우 기본값 설정
    end
end

% disp('Updated M matrix:');
% disp(M);

B = B * M;

% disp('B = ')
% disp(B)

disp('state_derivative = ');
disp(state_derivative);

disp('A * dx + B * du = ');
disp(A * dx + B * du);

error = state_derivative - (A * dx + B * du); %error : 3by1
disp('error = ');
disp(error);

if (error == 0)
    
    disp('error is zero');
    FCM = 1;
    FCMW = 1;
    avg_array_FCM = avg_array_FCM_;
    return

else
    del_uc = (inv(B)) * error; % del_uc는 3x1


    rotorMapping = rotorMapping'; % 이건 필수인듯?
    % disp('rotorMapping = ')
    % disp(rotorMapping(1,:))



    % error의 부호를 계산
    for i = 1:length(error)

        signError = sign(error(i));
        % disp('signError = ')
        % disp(signError)

        signMask = signError .* rotorMapping(i,:); % sign(error)를 대체
        % disp('signMask = ')
        % disp(signMask)

        for j = 1:length(signMask)
            if signMask(j) < 0
                refOmega(j) = omega_max; % signMask가 0보다 작으면 omega_max 할당
            else
                refOmega(j) = 0;         % signMask가 0 이상이면 0 할당
            end
        end

        % disp('refOmega = ');
        % disp(refOmega);

        % disp('omegaMotorSpeed = ');
        % disp(omegaMotorSpeed);

        maxDiff = abs(abs(omegaMotorSpeed) - refOmega); %maxDiff  8by1
        % disp('maxDiff = ')
        % disp(maxDiff)

        % Δu_MAX
        del_umax(i,1) = dt * (1/tau) * sum(maxDiff);
    end


    disp('abs(del_uc) = ')
    disp(abs(del_uc))

    disp('del_umax = ');
    disp(del_umax);


    controllability_matrix = ctrb(A,B);
    % disp('controllability_matrix = ')
    % disp(controllability_matrix)

    % 랭크 계산
    rank_con = rank(controllability_matrix);


    % disp('rank_con = ');
    % disp(rank_con);

    n = length(A);

    % disp('n = ')
    % disp(size(n))

    if rank_con < n || any(del_umax < abs(del_uc))
        FCM = 0;
    else
        FCM = 1;
    end

    [FCMW_, avg_array_FCM_] = calculate_FCMW(FCM,window_size_);

    FCMW = FCMW_;
    avg_array_FCM = avg_array_FCM_;

end % if end

disp('-----------------');

end

== matlab function FCMW/Subsystem2/MATLAB Function1 ==
  data: state_x_k input; estimation output; U_k input; K_store output; upper_bound output; lower_bound output
function [estimation, K_store,upper_bound, lower_bound]  = fcn(state_x_k, U_k)

%% Extended Kalman Filter Example
%% Initial Conditions
coder.extrinsic('delft_evaluate_jacobians');
coder.extrinsic('size');
coder.extrinsic('norm');
coder.extrinsic('eye');
coder.extrinsic('diag');
coder.extrinsic('subs');
coder.extrinsic('calculate_dynamics');
% persistent 변수 선언
persistent initialized xp Pp;

% 초기화가 필요할 때만 실행
if isempty(initialized)
    initialized = true; % 초기화 완료 표시
    xp = state_x_k;    % guess of initial posteriori estimation
    Pp = 100*eye(3); % guess of initial error covariance
    sigma_Pp = sqrt(diag(Pp));
    three_sigma = zeros(3,1);
    upper_bound = zeros(3,1);
    lower_bound = zeros(3,1);

    P = zeros(3,3);


    x_ = zeros(3,1);
    P_ = zeros(3,3);
    Pp_ = zeros(3,3);
    F = zeros(3,3);
    Q = zeros(3,3);
    R = zeros(3,3);
    K = zeros(3,3);
    H = zeros(3,3);
    I = zeros(3,3);
    estimation = zeros(3,1);
    K_store = zeros(1,1);
    disp('initialized.');
end

p = xp(1);
q = xp(2);
r = xp(3);

u_p = U_k(1);
u_q = U_k(2);
u_r = U_k(3);

sigma_w = 0.1;      % system noise (std of acceleration)
sigma_v = 0.2;      % measurement noise (std of position sensor)
Q = diag([sigma_w^2 sigma_w^2 sigma_w^2]); % system noise covariance matrix
R = diag([sigma_v^2 sigma_v^2 sigma_v^2]); % measurement noise covariance matrix
%% Dynamics
% system matrix

Gamma = [1 0 0;0 1 0;0 0 1];      % Gamma (related to system noise)
H = [1 0 0;0 1 0;0 0 1];          % Measurement matrix

%% KF Routine
    %% True dynamics
    % x(:,i+1) = [sin(x(2,i)*(i)) + randn*sigma_w; x(2,i) ]; % system dynamics
    % x = double(subs(F, {'p', 'q', 'r','u_p', 'u_q', 'u_r'},{p, q, r, u_p, u_q, u_r}));
    %% ====================================================
    %% Time update
    %% ====================================================
    %% Equation 1: Prediction of state
    % x_ = [sin(xp(2,i)*(i)); xp(2,i)];
    x_ = calculate_dynamics(p, q, r, u_p, u_q, u_r);
    %% compute Jacobian
    % F = [0 (i)*cos(x_(2)*(i));
    %     0 1];
    [F_, G_] = delft_evaluate_jacobians(p, q, r, u_p, u_q, u_r);
    %% Equation 2: Prediction of covariance
    F = F_;
    Pp_ = Pp;
    P_ = F*Pp_*F' + Gamma*Q*Gamma';
    %% ====================================================
    %% Measurement update
    %% ====================================================
    %% measurement generation
    % y(i) = H*x(:,i+1) + randn*sigma_v;
    y = state_x_k;
    %% Equation 3: Innovation Covariance
    S = H*P_*H'+R;
    %% Equation 4:  Residual
    nu = y-H*x_;
    %% Equation 5: Kalman gain
    K = P_*H'*S^-1;
    %% Equation 6: State update
    xp = x_ + K * nu;
    estimation = xp;
    %% Equation 7: Covariance update
    I = eye(size(K*H));
    Pp = (I-K*H)*P_;
    %% =====================================================
    %% storing error covariance for ploting
    sigma_Pp = sqrt(diag(Pp));
    % disp('sigma_Pp');
    % disp(size(sigma_Pp));
    three_sigma = 3 * sigma_Pp;
    upper_bound = xp + three_sigma;
    lower_bound = xp - three_sigma;
    %% storing Kalman gain for ploting
    K_store = norm(K);


    
%     %% Plot: position estimate x_1
% figure(1); clf; hold on;
% plot(t,x(1,:),'-b');                  % plot the real plant behavior
% plot(t(1:end-1),y,'.m');                       % plot the observations over this plant
% plot(t,xp(1,:),'-r');                 % plot the Kalman filter prediction over the plant
% plot(t,xp(1,:)+3*sigma_Pp(1,:),':k');  % The threshold in which the true state is
% plot(t,xp(1,:)-3*sigma_Pp(1,:),':k');
% xlabel('time, s'); ylabel('x1: m')
% legend('real','observation','KF','threshold')
% axis([-inf inf -10 10])
% %% Plot: velocity estimate x_2
% figure(2); clf; hold on;
% plot(t,x(2,:),'-b');                  % plot the real plant behavior
% plot(t,xp(2,:),'-r');                 % plot the Kalman filter prediction over the plant
% plot(t,xp(2,:)+3*sigma_Pp(2,:),':k');   % These two are the threshold in witch I'm certain that the plant state is at a given time
% plot(t,xp(2,:)-3*sigma_Pp(2,:),':k');
% xlabel('time, s'); ylabel('x2: rad/s')
% legend('true','KF','threshold')
% axis([-inf inf -5 20])
% %% Plot: Kalman gain norm
% figure(3);
% plot(t(1:end-1),K_store);
% xlabel('time, s'); ylabel('Kalman gain norm')

end

== matlab function FCMW/MATLAB Function1 ==
  data: gyroscopic_effect output; OMEGA_B input; phithetapsi input; omegaMotorSpeed input
function gyroscopic_effect = fcn(OMEGA_B, phithetapsi, omegaMotorSpeed)

coder.extrinsic('RotMat');
coder.extrinsic('cross');
coder.extrinsic('size');

% OMEGA_B : 3by1
p = OMEGA_B(1);
q = OMEGA_B(2);
r = OMEGA_B(3);
% disp('OMEGA_B = ');
% disp(size(OMEGA_B))

phi = phithetapsi(1);
theta = phithetapsi(2);
psi = phithetapsi(3);

ga = zeros(3, 1); % 각 로터에 대한 자이로스코픽 모멘트 저장
e_z_hat = [0;0;1]; % 가제보 좌표를 기반으로 z축의 unit vector
J_p = [1.545e-05 0 0;0 7.3574e-04 0;0 0 7.4861e-04]; % the moment of inertia related to 3 axes of body frame
% J_p = [0.001 0 0;0 0.001 0;0 0 0.006];

% e_z_hat : the unit vector in the inertial z axis
% e_3_hat : the unit vector in the body z axis : 3by1
e_3_hat = RotMat(phi, theta, psi, 8) * e_z_hat;  


% 부호 배열 (로터 방향에 따른 부호), Cq의 부호 사용
signs = [-1; -1; 1; 1; 1; 1; -1; -1];

% 자이로스코픽 효과 계산
% cross(OMEGA_B, e_3_hat) : 3by1
% sum(signs .* abs(omegaMotorSpeed)) : 1by1
% ga : 3by1
ga = J_p * cross(OMEGA_B, e_3_hat) * sum(signs .* abs(omegaMotorSpeed));
gyroscopic_effect = ga;

== matlab function FCMW/central difference ==
  data: p input; p_dot output; q input; r input; q_dot output; r_dot output
function [p_dot, q_dot, r_dot] = fcn(p, q, r)
    % 중앙 차분법으로 p_dot, q_dot, r_dot 계산
    % 그런데 중앙차분할때 미래의 데이터를 알아야하는데 알수가 없기 때문에 여기서 얻는 중앙차분값은 한스텦 이전의 상태에서의 미분값이다.

    % 상태 유지 변수
    persistent data_p data_q data_r dt initialized;

    % 초기화
    if isempty(initialized)
        data_p = zeros(3, 1); % 고정된 크기의 배열
        data_q = zeros(3, 1);
        data_r = zeros(3, 1);
        dt = 0.1; % 샘플링 간격
        initialized = true;
    end

    % FIFO 방식으로 데이터 업데이트
    data_p = [data_p(2:end); p]; % 가장 오래된 데이터 제거 후 새로운 데이터 추가
    data_q = [data_q(2:end); q];
    data_r = [data_r(2:end); r];

    % 중앙 차분법 적용 (배열 크기가 3인 경우)
    p_dot = (data_p(3) - data_p(1)) / (2 * dt); % 중앙 차분
    q_dot = (data_q(3) - data_q(1)) / (2 * dt); % 중앙 차분
    r_dot = (data_r(3) - data_r(1)) / (2 * dt); % 중앙 차분

    disp("data_p = ");
    disp(data_p);
end

== matlab function FCMW/MotorForceCalculation/octo geometricCalc ==
  data: L1 input; C output; L2 input; L3 input; b input; d input; C_pseudo_inverse output
function [C,C_pseudo_inverse] = geometricCalc(L1,L2,L3,b,d)

% k= (1/sqrt(2));

% C : control matrix
% C+ : pseudo-inverse
% u* : pseudo input
% u : input
% u = C x u*
% b = b*100; %왜냐하면 px4에는 로터속도가 210인데, 내가 얻는 속도는 21이기 때문이다. 그리고 모터 속도를 제곱해서 구하기때문에 10배차이*10배차이 = 100이다
% d = d*100; %왜냐하면 px4에는 로터속도가 210인데, 내가 얻는 속도는 21이기 때문이다. 그리고 모터 속도를 제곱해서 구하기때문에 10배차이*10배차이 = 100이다

C = [ -b,  -b,  -b,  -b,  -b,  -b,  -b,  -b;
     -b*L1,  b*L1, -b*L1,  -b*L1,  b*L1, b*L1,  b*L1, -b*L1;
     b*L3,  -b*L3, b*L2,  -b*L3,  b*L3, -b*L2,  b*L2,  -b*L2;
      -d,  -d, d, d, d, d, -d, -d ];

C_pseudo_inverse = pinv(C);


end

== matlab function FCMW/MATLAB Function3 ==
  data: Central_M_B output; p_dot input; q_dot input; r_dot input; p input; q input; r input
function Central_M_B = fcn(p_dot,q_dot,r_dot,p,q,r)

% 한스텦 이전의 미분값 과 한스텦 이전의 상태 값을 이용하여 MB 계산

I_v = [7.46 0 0;0 1.53 0;0 0 8.89];

Central_M_B = I_v * [p_dot;q_dot;r_dot] + cross([p;q;r] , I_v * [p;q;r]);

== matlab function FCMW/MotorForceCalculation/motorForceMomentCalc ==
  settings: updateMethod=DISCRETE
  data: omegaMotorSpeed input; f_t output; tau_B output; C input
function [f_t,tau_B] = motorForceMomentCalc(omegaMotorSpeed,C)

% FB = [fx; fy; fz];
% MB = [mx; my; mz];


% persistent 변수 선언
persistent is_initialized;

% 초기화가 필요할 때만 실행
if isempty(is_initialized)
    % 임시 변수에 초기화
    is_initialized = true;
end

FB_temp = zeros(3, 1);
MB_temp = zeros(3, 1);

% C : 4by8
% omegaMotor : 8by1
% actual_force_and_moment_acting_on_the_body = [ft; tau_x; tau_y; tau_z]'
actual_force_and_moment_acting_on_the_body = C * (abs(omegaMotorSpeed) .* abs(omegaMotorSpeed));
% actual_force_and_moment_acting_on_the_body = C * abs(omegaMotorSpeed);
disp('omegaMotor = ')
disp(abs(omegaMotorSpeed))
disp('omegaMotor.^2 = ')
disp(abs(omegaMotorSpeed) .* abs(omegaMotorSpeed))

FB_temp(1) = 0;
FB_temp(2) = 0;
FB_temp(3) = actual_force_and_moment_acting_on_the_body(1); % 추력 (Thrust)
MB_temp(1) = actual_force_and_moment_acting_on_the_body(2); % 롤 모멘트 (Roll moment)
MB_temp(2) = -actual_force_and_moment_acting_on_the_body(3); % 피치 모멘트 (Pitch moment)
MB_temp(3) = -actual_force_and_moment_acting_on_the_body(4); % 요 모멘트 (Yaw moment)

% 계산 결과를 출력 변수에 할당
f_t = FB_temp;
tau_B = MB_temp;


end
